simulink model "Rm1"  (Simulink 7.8)
settings: Solver=FixedStepDiscrete  StartTime=0.0  StopTime=10.0  RelTol=1e-3  SampleTimeConstraint=STIndependent
libraries: ApplFwS1v1_LIB x5
settings Model: Creator=z0035ypc  LastModifiedBy=z003019m
settings OptimizationCC: BooleanDataType=off  InlineParams=on
settings DebuggingCC: InheritedTsInSrcMsg=none  UnconnectedInputMsg=none  UnconnectedOutputMsg=none

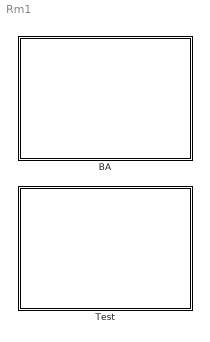
== system Rm1 ==
  BA : Subsystem
      mask Display: disp ('BA-Model');
  Test : Subsystem
      mask Display: disp ('Chart');

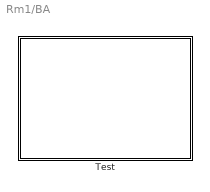
== system Rm1/BA ==
  Test : Subsystem
      mask Display: disp ('ViewNode Function');

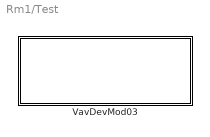
== system Rm1/Test ==
  VavDevMod03 : Subsystem
      mask Display: plot([0.5,0.5],[0.05,0.9]);text(0.5, 0.95,'VavDevMod03', 'HorizontalAlignment','center','VerticalAlignment','middle')

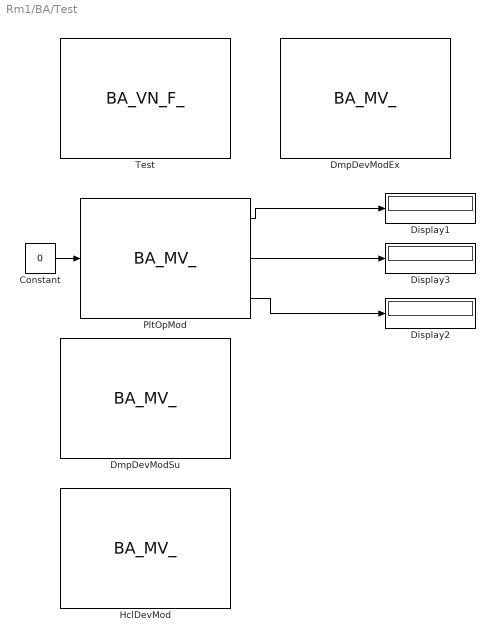
== system Rm1/BA/Test ==
  Constant : Constant  Value=0
  Display1 : Display
  Display2 : Display
  Display3 : Display
  DmpDevModEx : ApplFwS1v1_LIB/BA_OBJECT/BA_MV_  DefValue=1  NumOfStates=5  DeviceId=4194303  ObjectId=79691783
  DmpDevModSu : ApplFwS1v1_LIB/BA_OBJECT/BA_MV_  DefValue=1  NumOfStates=5  DeviceId=4194303  ObjectId=79691784
  HclDevMod : ApplFwS1v1_LIB/BA_OBJECT/BA_MV_  DefValue=1  NumOfStates=4  DeviceId=4194303  ObjectId=79691787
  PltOpMod : ApplFwS1v1_LIB/BA_OBJECT/BA_MV_  DefValue=1  NumOfStates=17  DeviceId=4194303  ObjectId=79691786
  Test : ApplFwS1v1_LIB/BA_OBJECT/BA_VN_F_  ItemDeviceId=[4194303 4194303 4194303 4194303]  ItemObjectId=[79691786 79691784 79691787 79691783]  DeviceId=[4194303]  ObjectId=[121634820]
  wires:
  PltOpMod/1 -> Display1/1
  PltOpMod/3 -> Display2/1
  PltOpMod/2 -> Display3/1
  Constant/1 -> PltOpMod/1

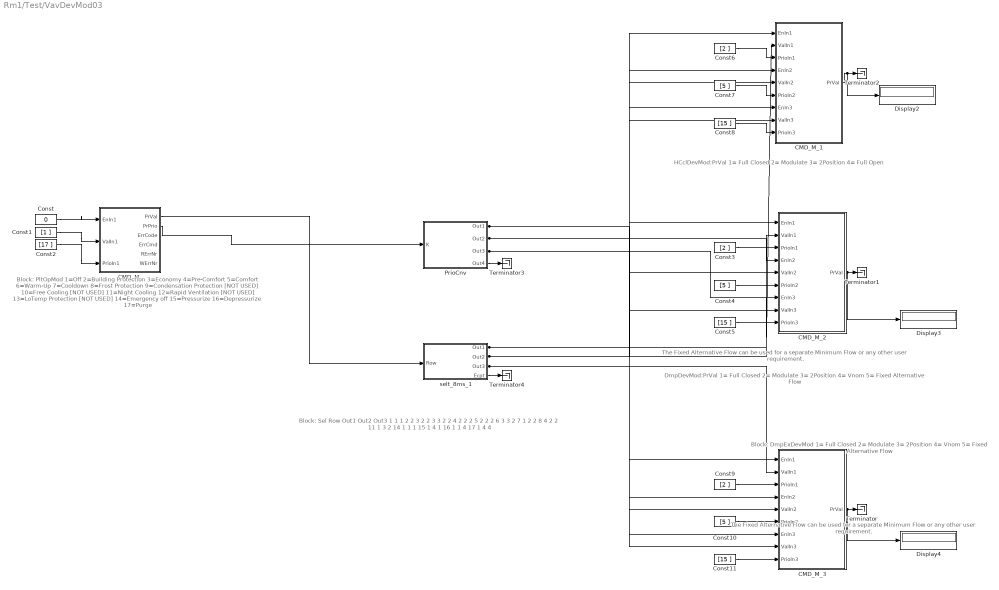
== system Rm1/Test/VavDevMod03 ==
  note: The Fixed Alternative Flow can be used for a separate Minimum Flow or any other user requirement.
  note: DmpDevMod:PrVal
      | 1= Full Closed
      | 2= Modulate
      | 3= 2Position
      | 4= Vnom
      | 5= Fixed Alternative Flow
  note: HCclDevMod:PrVal
      | 1= Full Closed
      | 2= Modulate
      | 3= 2Position
      | 4= Full Open
  note: Block: PltOpMod
      |
      | 1=Off
      | 2=Building Protection
      | 3=Economy
      | 4=Pre-Comfort
      | 5=Comfort
      | 6=Warm-Up
      | 7=Cooldown
      | 8=Frost Protection
      | 9=Condensation Protection [NOT USED]
      | 10=Free Cooling [NOT USED]
      | 11=Night Cooling
      | 12=Rapid Ventilation [NOT USED]
      | 13=LoTemp Protection [NOT USED]
      | 14=Emergency off
      | 15=Pressurize
      | 16=Depressurize
      | 17=Purge
  note: Block: Sel
      | Row  Out1  Out2   Out3
      | 1         1         1          2
      | 2         3         2          2
      | 3         3         2          2
      | 4         2         2          2
      | 5         2         2          2
      | 6         3         3          2
      | 7         1         2          2
      | 8         4         2          2
      | 11       1         3          2
      | 14       1         1          1
      | 15       1         4          1
      | 16       1         1          4
      | 17       1         4          4
  note: The Fixed Alternative Flow can be used for a separate Minimum Flow or any other user requirement.
  note: Block: DmpExDevMod
      | 1= Full Closed
      | 2= Modulate
      | 3= 2Position
      | 4= Vnom
      | 5= Fixed Alternative Flow
  CMD_M_ : Subsystem  mask{Invisible_1=off, Invisible_2=off, Invisible_3=off, Invisible_4=on, Invisible_5=on, Invisible_6=on, Invisible_7=on, Invisible_8=on, Invisible_9=on, Invisible_10=on, Invisible_11=on, Invisible_12=on, Invisible_13=on, Invisible_14=on, Invisible_15=on, Invisible_16=on, Invisible_17=off, Invisible_18=on, Invisible_19=off, Invisible_20=off, Invisible_21=off, Invisible_22=off, Invisible_23=off, Default_EnIn1=0, Default_ValIn1=0, Default_PrioIn1=0, Default_RptcIn1=0, Default_EnIn2=0, Default_ValIn2=0, Default_PrioIn2=0, Default_RptcIn2=0, Default_EnIn3=0, Default_ValIn3=0, Default_PrioIn3=0, Default_RptcIn3=0, Default_EnIn4=0, Default_ValIn4=0, Default_PrioIn4=0, Default_RptcIn4=0, DeviceId=4194303, ObjectId=121634820, ItemId=1, '=}
      mask prompts: Invisible_1 "EnIn1: Invisible"; Invisible_2 "ValIn1: Invisible"; Invisible_3 "PrioIn1: Invisible"; Invisible_4 "RptcIn1: Invisible"; Invisible_5 "EnIn2: Invisible"; Invisible_6 "ValIn2: Invisible"; Invisible_7 "PrioIn2: Invisible"; Invisible_8 "RptcIn2: Invisible"; Invisible_9 "EnIn3: Invisible"; Invisible_10 "ValIn3: Invisible"; Invisible_11 "PrioIn3: Invisible"; Invisible_12 "RptcIn3: Invisible"; Invisible_13 "EnIn4: Invisible"; Invisible_14 "ValIn4: Invisible"; Invisible_15 "PrioIn4: Invisible"; Invisible_16 "RptcIn4: Invisible"; Invisible_17 "PrVal: Invisible"; Invisible_18 "Valid: Invisible"; Invisible_19 "PrPrio: Invisible"; Invisible_20 "ErrCode: Invisible"; Invisible_21 "ErrCmd: Invisible"; Invisible_22 "RErrNr: Invisible"; Invisible_23 "WErrNr: Invisible"; Default_EnIn1 "EnIn1: Default"; Default_ValIn1 "ValIn1: Default"; Default_PrioIn1 "PrioIn1: Default"; Default_RptcIn1 "RptcIn1: Default"; Default_EnIn2 "EnIn2: Default"; Default_ValIn2 "ValIn2: Default"; Default_PrioIn2 "PrioIn2: Default"; Default_RptcIn2 "RptcIn2: Default"; Default_EnIn3 "EnIn3: Default"; Default_ValIn3 "ValIn3: Default"; Default_PrioIn3 "PrioIn3: Default"; Default_RptcIn3 "RptcIn3: Default"; Default_EnIn4 "EnIn4: Default"; Default_ValIn4 "ValIn4: Default"; Default_PrioIn4 "PrioIn4: Default"; Default_RptcIn4 "RptcIn4: Default"; DeviceId "BaObjRef.DeviceId"; ObjectId "BaObjRef.ObjectId"; ItemId "BaObjRef.ItemId"
      mask Help: web(['file:///' which('SiemensBuildingLibraryHelp0deDE.chm')])
      mask CallbackString: Callback(1)|Callback(2)|Callback(3)|Callback(4)|Callback(5)|Callback(6)|Callback(7)|Callback(8)|Callback(9)|Callback(10)|Callback(11)|Callback(12)|Callback(13)|Callback(14)|Callback(15)|Callback(16)|Callback(17)|Callback(18)|Callback(19)|Callback(20)|Callback(21)|Callback(22)|Callback(23)|Callback(24)|Callback(25)|Callback(26)|Callback(27)|Callback(28)|Callback(29)|Callback(30)|Callback(31)|Callback(32)|Callback(33)|Callback(34)|Callback(35)|Callback(36)|Callback(37)|Callback(38)|Callback(39)|||
      mask Display:
      | plot([0.5,0.5],[0,0.9])
      | text(0.5, 0.95,' CMD_M ', 'HorizontalAlignment', 'center')
  CMD_M_1 : Subsystem  mask{Invisible_1=off, Invisible_2=off, Invisible_3=off, Invisible_4=on, Invisible_5=off, Invisible_6=off, Invisible_7=off, Invisible_8=on, Invisible_9=off, Invisible_10=off, Invisible_11=off, Invisible_12=on, Invisible_13=on, Invisible_14=on, Invisible_15=on, Invisible_16=on, Invisible_17=off, Invisible_18=on, Invisible_19=on, Invisible_20=on, Invisible_21=on, Invisible_22=on, Invisible_23=on, Default_EnIn1=0, Default_ValIn1=0, Default_PrioIn1=0, Default_RptcIn1=0, Default_EnIn2=0, Default_ValIn2=0, Default_PrioIn2=0, Default_RptcIn2=0, Default_EnIn3=0, Default_ValIn3=0, Default_PrioIn3=0, Default_RptcIn3=0, Default_EnIn4=0, Default_ValIn4=0, Default_PrioIn4=0, Default_RptcIn4=0, DeviceId=4194303, ObjectId=121634820, ItemId=3, '=}
      mask prompts: Invisible_1 "EnIn1: Invisible"; Invisible_2 "ValIn1: Invisible"; Invisible_3 "PrioIn1: Invisible"; Invisible_4 "RptcIn1: Invisible"; Invisible_5 "EnIn2: Invisible"; Invisible_6 "ValIn2: Invisible"; Invisible_7 "PrioIn2: Invisible"; Invisible_8 "RptcIn2: Invisible"; Invisible_9 "EnIn3: Invisible"; Invisible_10 "ValIn3: Invisible"; Invisible_11 "PrioIn3: Invisible"; Invisible_12 "RptcIn3: Invisible"; Invisible_13 "EnIn4: Invisible"; Invisible_14 "ValIn4: Invisible"; Invisible_15 "PrioIn4: Invisible"; Invisible_16 "RptcIn4: Invisible"; Invisible_17 "PrVal: Invisible"; Invisible_18 "Valid: Invisible"; Invisible_19 "PrPrio: Invisible"; Invisible_20 "ErrCode: Invisible"; Invisible_21 "ErrCmd: Invisible"; Invisible_22 "RErrNr: Invisible"; Invisible_23 "WErrNr: Invisible"; Default_EnIn1 "EnIn1: Default"; Default_ValIn1 "ValIn1: Default"; Default_PrioIn1 "PrioIn1: Default"; Default_RptcIn1 "RptcIn1: Default"; Default_EnIn2 "EnIn2: Default"; Default_ValIn2 "ValIn2: Default"; Default_PrioIn2 "PrioIn2: Default"; Default_RptcIn2 "RptcIn2: Default"; Default_EnIn3 "EnIn3: Default"; Default_ValIn3 "ValIn3: Default"; Default_PrioIn3 "PrioIn3: Default"; Default_RptcIn3 "RptcIn3: Default"; Default_EnIn4 "EnIn4: Default"; Default_ValIn4 "ValIn4: Default"; Default_PrioIn4 "PrioIn4: Default"; Default_RptcIn4 "RptcIn4: Default"; DeviceId "BaObjRef.DeviceId"; ObjectId "BaObjRef.ObjectId"; ItemId "BaObjRef.ItemId"
      mask Help: web(['file:///' which('SiemensBuildingLibraryHelp0deDE.chm')])
      mask CallbackString: Callback(1)|Callback(2)|Callback(3)|Callback(4)|Callback(5)|Callback(6)|Callback(7)|Callback(8)|Callback(9)|Callback(10)|Callback(11)|Callback(12)|Callback(13)|Callback(14)|Callback(15)|Callback(16)|Callback(17)|Callback(18)|Callback(19)|Callback(20)|Callback(21)|Callback(22)|Callback(23)|Callback(24)|Callback(25)|Callback(26)|Callback(27)|Callback(28)|Callback(29)|Callback(30)|Callback(31)|Callback(32)|Callback(33)|Callback(34)|Callback(35)|Callback(36)|Callback(37)|Callback(38)|Callback(39)|||
      mask Display:
      | plot([0.5,0.5],[0,0.9])
      | text(0.5, 0.95,' CMD_M ', 'HorizontalAlignment', 'center')
  CMD_M_2 : Subsystem  mask{Invisible_1=off, Invisible_2=off, Invisible_3=off, Invisible_4=on, Invisible_5=off, Invisible_6=off, Invisible_7=off, Invisible_8=on, Invisible_9=off, Invisible_10=off, Invisible_11=off, Invisible_12=on, Invisible_13=on, Invisible_14=on, Invisible_15=on, Invisible_16=on, Invisible_17=off, Invisible_18=on, Invisible_19=on, Invisible_20=on, Invisible_21=on, Invisible_22=on, Invisible_23=on, Default_EnIn1=0, Default_ValIn1=0, Default_PrioIn1=0, Default_RptcIn1=0, Default_EnIn2=0, Default_ValIn2=0, Default_PrioIn2=0, Default_RptcIn2=0, Default_EnIn3=0, Default_ValIn3=0, Default_PrioIn3=0, Default_RptcIn3=0, Default_EnIn4=0, Default_ValIn4=0, Default_PrioIn4=0, Default_RptcIn4=0, DeviceId=4194303, ObjectId=121634820, ItemId=2, '=}
      mask prompts: Invisible_1 "EnIn1: Invisible"; Invisible_2 "ValIn1: Invisible"; Invisible_3 "PrioIn1: Invisible"; Invisible_4 "RptcIn1: Invisible"; Invisible_5 "EnIn2: Invisible"; Invisible_6 "ValIn2: Invisible"; Invisible_7 "PrioIn2: Invisible"; Invisible_8 "RptcIn2: Invisible"; Invisible_9 "EnIn3: Invisible"; Invisible_10 "ValIn3: Invisible"; Invisible_11 "PrioIn3: Invisible"; Invisible_12 "RptcIn3: Invisible"; Invisible_13 "EnIn4: Invisible"; Invisible_14 "ValIn4: Invisible"; Invisible_15 "PrioIn4: Invisible"; Invisible_16 "RptcIn4: Invisible"; Invisible_17 "PrVal: Invisible"; Invisible_18 "Valid: Invisible"; Invisible_19 "PrPrio: Invisible"; Invisible_20 "ErrCode: Invisible"; Invisible_21 "ErrCmd: Invisible"; Invisible_22 "RErrNr: Invisible"; Invisible_23 "WErrNr: Invisible"; Default_EnIn1 "EnIn1: Default"; Default_ValIn1 "ValIn1: Default"; Default_PrioIn1 "PrioIn1: Default"; Default_RptcIn1 "RptcIn1: Default"; Default_EnIn2 "EnIn2: Default"; Default_ValIn2 "ValIn2: Default"; Default_PrioIn2 "PrioIn2: Default"; Default_RptcIn2 "RptcIn2: Default"; Default_EnIn3 "EnIn3: Default"; Default_ValIn3 "ValIn3: Default"; Default_PrioIn3 "PrioIn3: Default"; Default_RptcIn3 "RptcIn3: Default"; Default_EnIn4 "EnIn4: Default"; Default_ValIn4 "ValIn4: Default"; Default_PrioIn4 "PrioIn4: Default"; Default_RptcIn4 "RptcIn4: Default"; DeviceId "BaObjRef.DeviceId"; ObjectId "BaObjRef.ObjectId"; ItemId "BaObjRef.ItemId"
      mask Help: web(['file:///' which('SiemensBuildingLibraryHelp0deDE.chm')])
      mask CallbackString: Callback(1)|Callback(2)|Callback(3)|Callback(4)|Callback(5)|Callback(6)|Callback(7)|Callback(8)|Callback(9)|Callback(10)|Callback(11)|Callback(12)|Callback(13)|Callback(14)|Callback(15)|Callback(16)|Callback(17)|Callback(18)|Callback(19)|Callback(20)|Callback(21)|Callback(22)|Callback(23)|Callback(24)|Callback(25)|Callback(26)|Callback(27)|Callback(28)|Callback(29)|Callback(30)|Callback(31)|Callback(32)|Callback(33)|Callback(34)|Callback(35)|Callback(36)|Callback(37)|Callback(38)|Callback(39)|||
      mask Display:
      | plot([0.5,0.5],[0,0.9])
      | text(0.5, 0.95,' CMD_M ', 'HorizontalAlignment', 'center')
  CMD_M_3 : Subsystem  mask{Invisible_1=off, Invisible_2=off, Invisible_3=off, Invisible_4=on, Invisible_5=off, Invisible_6=off, Invisible_7=off, Invisible_8=on, Invisible_9=off, Invisible_10=off, Invisible_11=off, Invisible_12=on, Invisible_13=on, Invisible_14=on, Invisible_15=on, Invisible_16=on, Invisible_17=off, Invisible_18=on, Invisible_19=on, Invisible_20=on, Invisible_21=on, Invisible_22=on, Invisible_23=on, Default_EnIn1=0, Default_ValIn1=0, Default_PrioIn1=0, Default_RptcIn1=0, Default_EnIn2=0, Default_ValIn2=0, Default_PrioIn2=0, Default_RptcIn2=0, Default_EnIn3=0, Default_ValIn3=0, Default_PrioIn3=0, Default_RptcIn3=0, Default_EnIn4=0, Default_ValIn4=0, Default_PrioIn4=0, Default_RptcIn4=0, DeviceId=4194303, ObjectId=121634820, ItemId=4, '=}
      mask prompts: Invisible_1 "EnIn1: Invisible"; Invisible_2 "ValIn1: Invisible"; Invisible_3 "PrioIn1: Invisible"; Invisible_4 "RptcIn1: Invisible"; Invisible_5 "EnIn2: Invisible"; Invisible_6 "ValIn2: Invisible"; Invisible_7 "PrioIn2: Invisible"; Invisible_8 "RptcIn2: Invisible"; Invisible_9 "EnIn3: Invisible"; Invisible_10 "ValIn3: Invisible"; Invisible_11 "PrioIn3: Invisible"; Invisible_12 "RptcIn3: Invisible"; Invisible_13 "EnIn4: Invisible"; Invisible_14 "ValIn4: Invisible"; Invisible_15 "PrioIn4: Invisible"; Invisible_16 "RptcIn4: Invisible"; Invisible_17 "PrVal: Invisible"; Invisible_18 "Valid: Invisible"; Invisible_19 "PrPrio: Invisible"; Invisible_20 "ErrCode: Invisible"; Invisible_21 "ErrCmd: Invisible"; Invisible_22 "RErrNr: Invisible"; Invisible_23 "WErrNr: Invisible"; Default_EnIn1 "EnIn1: Default"; Default_ValIn1 "ValIn1: Default"; Default_PrioIn1 "PrioIn1: Default"; Default_RptcIn1 "RptcIn1: Default"; Default_EnIn2 "EnIn2: Default"; Default_ValIn2 "ValIn2: Default"; Default_PrioIn2 "PrioIn2: Default"; Default_RptcIn2 "RptcIn2: Default"; Default_EnIn3 "EnIn3: Default"; Default_ValIn3 "ValIn3: Default"; Default_PrioIn3 "PrioIn3: Default"; Default_RptcIn3 "RptcIn3: Default"; Default_EnIn4 "EnIn4: Default"; Default_ValIn4 "ValIn4: Default"; Default_PrioIn4 "PrioIn4: Default"; Default_RptcIn4 "RptcIn4: Default"; DeviceId "BaObjRef.DeviceId"; ObjectId "BaObjRef.ObjectId"; ItemId "BaObjRef.ItemId"
      mask Help: web(['file:///' which('SiemensBuildingLibraryHelp0deDE.chm')])
      mask CallbackString: Callback(1)|Callback(2)|Callback(3)|Callback(4)|Callback(5)|Callback(6)|Callback(7)|Callback(8)|Callback(9)|Callback(10)|Callback(11)|Callback(12)|Callback(13)|Callback(14)|Callback(15)|Callback(16)|Callback(17)|Callback(18)|Callback(19)|Callback(20)|Callback(21)|Callback(22)|Callback(23)|Callback(24)|Callback(25)|Callback(26)|Callback(27)|Callback(28)|Callback(29)|Callback(30)|Callback(31)|Callback(32)|Callback(33)|Callback(34)|Callback(35)|Callback(36)|Callback(37)|Callback(38)|Callback(39)|||
      mask Display:
      | plot([0.5,0.5],[0,0.9])
      | text(0.5, 0.95,' CMD_M ', 'HorizontalAlignment', 'center')
  Const : Constant  Value=0  SampleTime=-1
  Const1 : Constant  Value=[1 ]  SampleTime=-1
  Const10 : Constant  Value=[5 ]  SampleTime=-1
  Const11 : Constant  Value=[15 ]  SampleTime=-1
  Const2 : Constant  Value=[17 ]  SampleTime=-1
  Const3 : Constant  Value=[2 ]  SampleTime=-1
  Const4 : Constant  Value=[5 ]  SampleTime=-1
  Const5 : Constant  Value=[15 ]  SampleTime=-1
  Const6 : Constant  Value=[2 ]  SampleTime=-1
  Const7 : Constant  Value=[5 ]  SampleTime=-1
  Const8 : Constant  Value=[15 ]  SampleTime=-1
  Const9 : Constant  Value=[2 ]  SampleTime=-1
  Display2 : Display
  Display3 : Display
  Display4 : Display
  PrioCnv : Subsystem  AncestorBlock=ApplFwS1v1_LIB/CONVERT/PRIO_CNV_  mask{Invisible_1=off, Invisible_2=on, Invisible_3=on, Invisible_4=on, Invisible_5=on, Invisible_6=on, Invisible_7=on, Invisible_8=on, Invisible_9=on, Invisible_10=on, Invisible_11=on, Invisible_12=on, Invisible_13=on, Invisible_14=on, Invisible_15=on, Invisible_16=on, Invisible_17=on, Invisible_18=on, Invisible_19=off, Invisible_20=off, Invisible_21=off, Invisible_22=off, Default_K=0, Default_Prio1=1, Default_Prio2=1, Default_Prio3=1, Default_Prio4=2, Default_Prio5=2, Default_Prio6=2, Default_Prio7=3, Default_Prio8=3, Default_Prio9=3, Default_Prio10=3, Default_Prio11=3, Default_Prio12=3, Default_Prio13=3, Default_Prio14=3, Default_Prio15=3, Default_Prio16=3, Default_Prio17=3, '=}
      mask prompts: Invisible_1 "K: Invisible"; Invisible_2 "Prio1: Invisible"; Invisible_3 "Prio2: Invisible"; Invisible_4 "Prio3: Invisible"; Invisible_5 "Prio4: Invisible"; Invisible_6 "Prio5: Invisible"; Invisible_7 "Prio6: Invisible"; Invisible_8 "Prio7: Invisible"; Invisible_9 "Prio8: Invisible"; Invisible_10 "Prio9: Invisible"; Invisible_11 "Prio10: Invisible"; Invisible_12 "Prio11: Invisible"; Invisible_13 "Prio12: Invisible"; Invisible_14 "Prio13: Invisible"; Invisible_15 "Prio14: Invisible"; Invisible_16 "Prio15: Invisible"; Invisible_17 "Prio16: Invisible"; Invisible_18 "Prio17: Invisible"; Invisible_19 "Out1: Invisible"; Invisible_20 "Out2: Invisible"; Invisible_21 "Out3: Invisible"; Invisible_22 "Out4: Invisible"; Default_K "K: Default"; Default_Prio1 "Prio1: Default"; Default_Prio2 "Prio2: Default"; Default_Prio3 "Prio3: Default"; Default_Prio4 "Prio4: Default"; Default_Prio5 "Prio5: Default"; Default_Prio6 "Prio6: Default"; Default_Prio7 "Prio7: Default"; Default_Prio8 "Prio8: Default"; Default_Prio9 "Prio9: Default"; Default_Prio10 "Prio10: Default"; Default_Prio11 "Prio11: Default"; Default_Prio12 "Prio12: Default"; Default_Prio13 "Prio13: Default"; Default_Prio14 "Prio14: Default"; Default_Prio15 "Prio15: Default"; Default_Prio16 "Prio16: Default"; Default_Prio17 "Prio17: Default"
      mask Help: web(['file:///' which('SiemensBuildingLibraryHelp0deDE.chm')])
      mask CallbackString: Callback(1)|Callback(2)|Callback(3)|Callback(4)|Callback(5)|Callback(6)|Callback(7)|Callback(8)|Callback(9)|Callback(10)|Callback(11)|Callback(12)|Callback(13)|Callback(14)|Callback(15)|Callback(16)|Callback(17)|Callback(18)|Callback(19)|Callback(20)|Callback(21)|Callback(22)|Callback(23)|Callback(24)|Callback(25)|Callback(26)|Callback(27)|Callback(28)|Callback(29)|Callback(30)|Callback(31)|Callback(32)|Callback(33)|Callback(34)|Callback(35)|Callback(36)|Callback(37)|Callback(38)|Callback(39)|Callback(40)
      mask Display:
      | plot([0.5,0.5],[0,0.9])
      | text(0.5, 0.95,' PRIO_CNV ', 'HorizontalAlignment', 'center')
  Terminator{,1..4} (5 alike) : Terminator
  selt_8ms_1 : Subsystem  AncestorBlock=ApplFwS1v1_LIB/MULTIPLX/SELT_8MS_  mask{Invisible_1=off, Invisible_2=on, Invisible_3=on, Invisible_4=on, Invisible_5=on, Invisible_6=on, Invisible_7=on, Invisible_8=on, Invisible_9=on, Invisible_10=on, Invisible_11=on, Invisible_12=on, Invisible_13=on, Invisible_14=on, Invisible_15=on, Invisible_16=on, Invisible_17=on, Invisible_18=on, Invisible_19=on, Invisible_20=on, Invisible_21=on, Invisible_22=on, Invisible_23=on, Invisible_24=on, Invisible_25=on, Invisible_26=on, Invisible_27=on, Invisible_28=off, Invisible_29=off, Invisible_30=off, Invisible_31=on, Invisible_32=on, Invisible_33=on, Invisible_34=on, Invisible_35=on, Invisible_36=off, Invisible_37=on, Default_Row=0, Default_RowCnd=[ 1 2 3 4 5 6 7 8 9 10 11 12 13 14 15 16 17 18 19 20 21 22 23 24 ], Default_ValRow1=[ 1 1 2 1 1 1 1 1 ], Default_ValRow2=[ 3 2 2 1 1 1 1 1 ], Default_ValRow3=[ 3 2 2 1 1 1 1 1 ], Default_ValRow4=[ 2 2 2 1 1 1 1 1 ], Default_ValRow5=[ 2 2 2 1 1 1 1 1 ], Default_ValRow6=[ 3 3 2 1 1 1 1 1 ], Default_ValRow7=[ 1 2 2 1 1 1 1 1 ], Default_ValRow8=[ 4 2 2 1 1 1 1 1 ], Default_ValRow9=[ 1 1 1 1 1 1 1 1 ], Default_ValRow10=[ 1 1 1 1 1 1 1 1 ], Default_ValRow11=[ 1 3 2 1 1 1 1 1 ], Default_ValRow12=[ 1 1 1 1 1 1 1 1 ], Default_ValRow13=[ 1 1 1 1 1 1 1 1 ], Default_ValRow14=[ 1 1 1 1 1 1 1 1 ], Default_ValRow15=[ 1 4 1 1 1 1 1 1 ], Default_ValRow16=[ 1 1 4 1 1 1 1 1 ], Default_ValRow17=[ 1 4 4 1 1 1 1 1 ], Default_ValRow18=[ 1 1 1 1 1 1 1 1 ], Default_ValRow19=[ 1 1 1 1 1 1 1 1 ], Default_ValRow20=[ 1 1 1 1 1 1 1 1 ], Default_ValRow21=[ 1 1 1 1 1 1 1 1 ], Default_ValRow22=[ 1 1 1 1 1 1 1 1 ], Default_ValRow23=[ 1 1 1 1 1 1 1 1 ], Default_ValRow24=[ 1 1 1 1 1 1 1 1 ], Default_EcptVal=1}
      mask prompts: Invisible_1 "Row: Invisible"; Invisible_2 "RowCnd: Invisible"; Invisible_3 "ValRow1: Invisible"; Invisible_4 "ValRow2: Invisible"; Invisible_5 "ValRow3: Invisible"; Invisible_6 "ValRow4: Invisible"; Invisible_7 "ValRow5: Invisible"; Invisible_8 "ValRow6: Invisible"; Invisible_9 "ValRow7: Invisible"; Invisible_10 "ValRow8: Invisible"; Invisible_11 "ValRow9: Invisible"; Invisible_12 "ValRow10: Invisible"; Invisible_13 "ValRow11: Invisible"; Invisible_14 "ValRow12: Invisible"; Invisible_15 "ValRow13: Invisible"; Invisible_16 "ValRow14: Invisible"; Invisible_17 "ValRow15: Invisible"; Invisible_18 "ValRow16: Invisible"; Invisible_19 "ValRow17: Invisible"; Invisible_20 "ValRow18: Invisible"; Invisible_21 "ValRow19: Invisible"; Invisible_22 "ValRow20: Invisible"; Invisible_23 "ValRow21: Invisible"; Invisible_24 "ValRow22: Invisible"; Invisible_25 "ValRow23: Invisible"; Invisible_26 "ValRow24: Invisible"; Invisible_27 "EcptVal: Invisible"; Invisible_28 "Out1: Invisible"; Invisible_29 "Out2: Invisible"; Invisible_30 "Out3: Invisible"; Invisible_31 "Out4: Invisible"; Invisible_32 "Out5: Invisible"; Invisible_33 "Out6: Invisible"; Invisible_34 "Out7: Invisible"; Invisible_35 "Out8: Invisible"; Invisible_36 "EcptActv: Invisible"; Invisible_37 "DataBlkItf: Invisible"; Default_Row "Row: Default"; Default_RowCnd "RowCnd: Default"; Default_ValRow1 "ValRow1: Default"; Default_ValRow2 "ValRow2: Default"; Default_ValRow3 "ValRow3: Default"; Default_ValRow4 "ValRow4: Default"; Default_ValRow5 "ValRow5: Default"; Default_ValRow6 "ValRow6: Default"; Default_ValRow7 "ValRow7: Default"; Default_ValRow8 "ValRow8: Default"; Default_ValRow9 "ValRow9: Default"; Default_ValRow10 "ValRow10: Default"; Default_ValRow11 "ValRow11: Default"; Default_ValRow12 "ValRow12: Default"; Default_ValRow13 "ValRow13: Default"; Default_ValRow14 "ValRow14: Default"; Default_ValRow15 "ValRow15: Default"; Default_ValRow16 "ValRow16: Default"; Default_ValRow17 "ValRow17: Default"; Default_ValRow18 "ValRow18: Default"; Default_ValRow19 "ValRow19: Default"; Default_ValRow20 "ValRow20: Default"; Default_ValRow21 "ValRow21: Default"; Default_ValRow22 "ValRow22: Default"; Default_ValRow23 "ValRow23: Default"; Default_ValRow24 "ValRow24: Default"; Default_EcptVal "EcptVal: Default"
      mask Help: web(['file:///' which('SiemensBuildingLibraryHelp0deDE.chm')])
      mask CallbackString: Callback(1)|Callback(2)|Callback(3)|Callback(4)|Callback(5)|Callback(6)|Callback(7)|Callback(8)|Callback(9)|Callback(10)|Callback(11)|Callback(12)|Callback(13)|Callback(14)|Callback(15)|Callback(16)|Callback(17)|Callback(18)|Callback(19)|Callback(20)|Callback(21)|Callback(22)|Callback(23)|Callback(24)|Callback(25)|Callback(26)|Callback(27)|Callback(28)|Callback(29)|Callback(30)|Callback(31)|Callback(32)|Callback(33)|Callback(34)|Callback(35)|Callback(36)|Callback(37)|Callback(38)|Callback(39)|Callback(40)|Callback(41)|Callback(42)|Callback(43)|Callback(44)|Callback(45)|Callback(46)|Callback(47)|Callback(48)|Callback(49)|Callback(50)|Callback(51)|Callback(52)|Callback(53)|Callback(54)|Callback(55)|Callback(56)|Callback(57)|Callback(58)|Callback(59)|Callback(60)|Callback(61)|Callback(62)|Callback(63)|Callback(64)
      mask Display:
      | plot([0.5,0.5],[0,0.9])
      | text(0.5, 0.95,' SELT_8MS ', 'HorizontalAlignment', 'center')
  wires:
  Const/1 -> CMD_M_/1(EnIn1)
  Const1/1 -> CMD_M_/2(ValIn1)
  Const2/1 -> CMD_M_/3(PrioIn1)
  Const3/1 -> CMD_M_2/3(PrioIn1)
  Const4/1 -> CMD_M_2/6(PrioIn2)
  Const5/1 -> CMD_M_2/9(PrioIn3)
  Const6/1 -> CMD_M_1/3(PrioIn1)
  Const7/1 -> CMD_M_1/6(PrioIn2)
  Const8/1 -> CMD_M_1/9(PrioIn3)
  Const9/1 -> CMD_M_3/3(PrioIn1)
  Const10/1 -> CMD_M_3/6(PrioIn2)
  Const11/1 -> CMD_M_3/9(PrioIn3)
  CMD_M_/1(PrVal) -> selt_8ms_1/1(Row)
  CMD_M_/2(PrPrio) -> PrioCnv/1(K)
  PrioCnv/1(Out1) -> CMD_M_1/1(EnIn1), CMD_M_2/1(EnIn1), CMD_M_3/1(EnIn1)
  PrioCnv/2(Out2) -> CMD_M_1/4(EnIn2), CMD_M_2/4(EnIn2), CMD_M_3/4(EnIn2)
  PrioCnv/3(Out3) -> CMD_M_1/7(EnIn3), CMD_M_2/7(EnIn3), CMD_M_3/7(EnIn3)
  selt_8ms_1/1(Out1) -> CMD_M_1/8(ValIn3), CMD_M_1/5(ValIn2), CMD_M_1/2(ValIn1)
  selt_8ms_1/2(Out2) -> CMD_M_2/8(ValIn3), CMD_M_2/5(ValIn2), CMD_M_2/2(ValIn1)
  selt_8ms_1/3(Out3) -> CMD_M_3/8(ValIn3), CMD_M_3/5(ValIn2), CMD_M_3/2(ValIn1)
  CMD_M_3/1(PrVal) -> Terminator/1, Display4/1
  CMD_M_2/1(PrVal) -> Terminator1/1, Display3/1
  CMD_M_1/1(PrVal) -> Terminator2/1, Display2/1
  PrioCnv/4(Out4) -> Terminator3/1
  selt_8ms_1/4(Ecpt) -> Terminator4/1

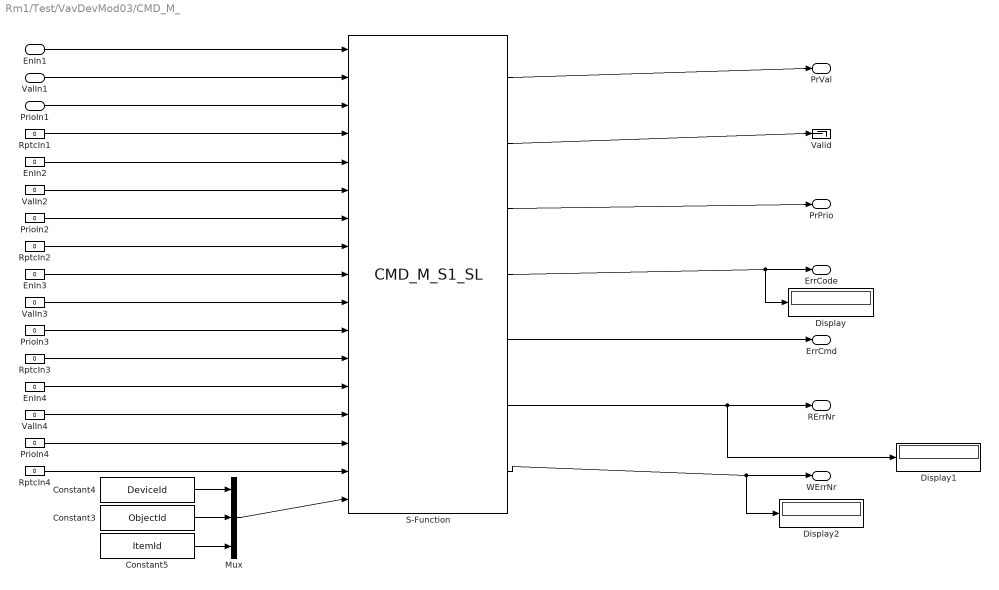
== system Rm1/Test/VavDevMod03/CMD_M_ ==
  EnIn1 : Inport
  ValIn1 : Inport  Port=2
  PrioIn1 : Inport  Port=3
  Constant3 : Constant  Value=ObjectId  OutDataTypeStr=Inherit: Inherit via back propagation  SampleTime=-1
  Constant4 : Constant  Value=DeviceId  OutDataTypeStr=Inherit: Inherit via back propagation  SampleTime=-1
  Constant5 : Constant  Value=ItemId  OutDataTypeStr=Inherit: Inherit via back propagation  SampleTime=-1
  Display : Display
  Display1 : Display
  Display2 : Display
  EnIn2 : Constant  Value=0  SampleTime=-1
  EnIn3 : Constant  Value=0  SampleTime=-1
  EnIn4 : Constant  Value=0  SampleTime=-1
  Mux : Mux  Inputs=3
  PrioIn2 : Constant  Value=0  SampleTime=-1
  PrioIn3 : Constant  Value=0  SampleTime=-1
  PrioIn4 : Constant  Value=0  SampleTime=-1
  RptcIn{1..4} (4 alike) : Constant  Value=0  SampleTime=-1
  S-Function : S-Function  FunctionName=CMD_M_S1_SL  Parameters=-1  EnableBusSupport=off
  ValIn2 : Constant  Value=0  SampleTime=-1
  ValIn3 : Constant  Value=0  SampleTime=-1
  ValIn4 : Constant  Value=0  SampleTime=-1
  Valid : Terminator
  PrVal : Outport
  PrPrio : Outport  Port=2
  ErrCode : Outport  Port=3
  ErrCmd : Outport  Port=4
  RErrNr : Outport  Port=5
  WErrNr : Outport  Port=6
  wires:
  EnIn1/1 -> S-Function/1
  ValIn1/1 -> S-Function/2
  PrioIn1/1 -> S-Function/3
  RptcIn1/1 -> S-Function/4
  EnIn2/1 -> S-Function/5
  ValIn2/1 -> S-Function/6
  PrioIn2/1 -> S-Function/7
  RptcIn2/1 -> S-Function/8
  EnIn3/1 -> S-Function/9
  ValIn3/1 -> S-Function/10
  PrioIn3/1 -> S-Function/11
  RptcIn3/1 -> S-Function/12
  EnIn4/1 -> S-Function/13
  ValIn4/1 -> S-Function/14
  PrioIn4/1 -> S-Function/15
  RptcIn4/1 -> S-Function/16
  Constant4/1 -> Mux/1
  Constant3/1 -> Mux/2
  Constant5/1 -> Mux/3
  Mux/1 -> S-Function/17
  S-Function/1 -> PrVal/1
  S-Function/2 -> Valid/1
  S-Function/3 -> PrPrio/1
  S-Function/4 -> ErrCode/1, Display/1
  S-Function/5 -> ErrCmd/1
  S-Function/6 -> Display1/1, RErrNr/1
  S-Function/7 -> WErrNr/1, Display2/1

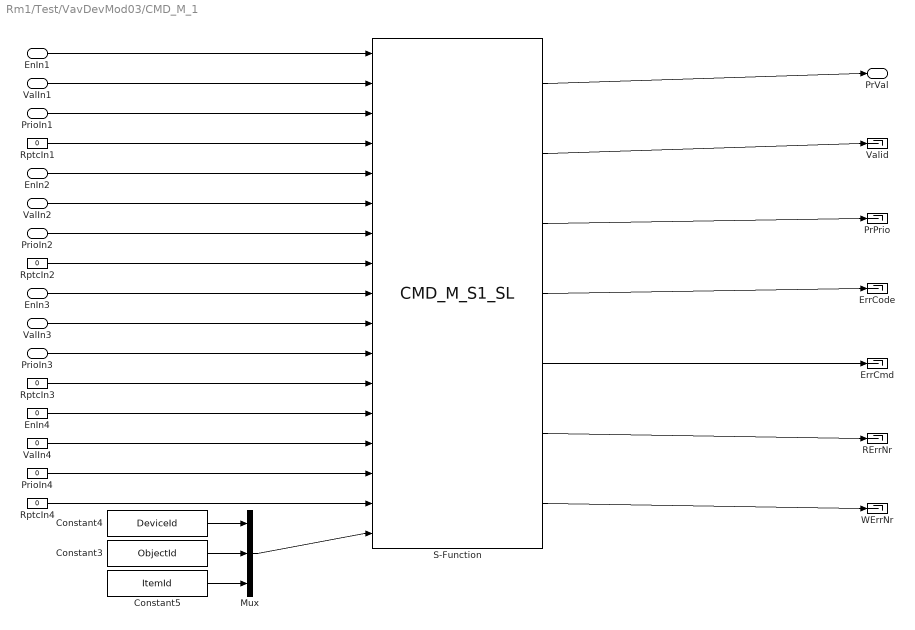
== system Rm1/Test/VavDevMod03/CMD_M_1 ==
  EnIn1 : Inport
  ValIn1 : Inport  Port=2
  PrioIn1 : Inport  Port=3
  EnIn2 : Inport  Port=4
  ValIn2 : Inport  Port=5
  PrioIn2 : Inport  Port=6
  EnIn3 : Inport  Port=7
  ValIn3 : Inport  Port=8
  PrioIn3 : Inport  Port=9
  Constant3 : Constant  Value=ObjectId  OutDataTypeStr=Inherit: Inherit via back propagation  SampleTime=-1
  Constant4 : Constant  Value=DeviceId  OutDataTypeStr=Inherit: Inherit via back propagation  SampleTime=-1
  Constant5 : Constant  Value=ItemId  OutDataTypeStr=Inherit: Inherit via back propagation  SampleTime=-1
  EnIn4 : Constant  Value=0  SampleTime=-1
  ErrCmd : Terminator
  ErrCode : Terminator
  Mux : Mux  Inputs=3
  PrPrio : Terminator
  PrioIn4 : Constant  Value=0  SampleTime=-1
  RErrNr : Terminator
  RptcIn{1..4} (4 alike) : Constant  Value=0  SampleTime=-1
  S-Function : S-Function  FunctionName=CMD_M_S1_SL  Parameters=-1  EnableBusSupport=off
  ValIn4 : Constant  Value=0  SampleTime=-1
  Valid : Terminator
  WErrNr : Terminator
  PrVal : Outport
  wires:
  EnIn1/1 -> S-Function/1
  ValIn1/1 -> S-Function/2
  PrioIn1/1 -> S-Function/3
  RptcIn1/1 -> S-Function/4
  EnIn2/1 -> S-Function/5
  ValIn2/1 -> S-Function/6
  PrioIn2/1 -> S-Function/7
  RptcIn2/1 -> S-Function/8
  EnIn3/1 -> S-Function/9
  ValIn3/1 -> S-Function/10
  PrioIn3/1 -> S-Function/11
  RptcIn3/1 -> S-Function/12
  EnIn4/1 -> S-Function/13
  ValIn4/1 -> S-Function/14
  PrioIn4/1 -> S-Function/15
  RptcIn4/1 -> S-Function/16
  Constant4/1 -> Mux/1
  Constant3/1 -> Mux/2
  Constant5/1 -> Mux/3
  Mux/1 -> S-Function/17
  S-Function/1 -> PrVal/1
  S-Function/2 -> Valid/1
  S-Function/3 -> PrPrio/1
  S-Function/4 -> ErrCode/1
  S-Function/5 -> ErrCmd/1
  S-Function/6 -> RErrNr/1
  S-Function/7 -> WErrNr/1

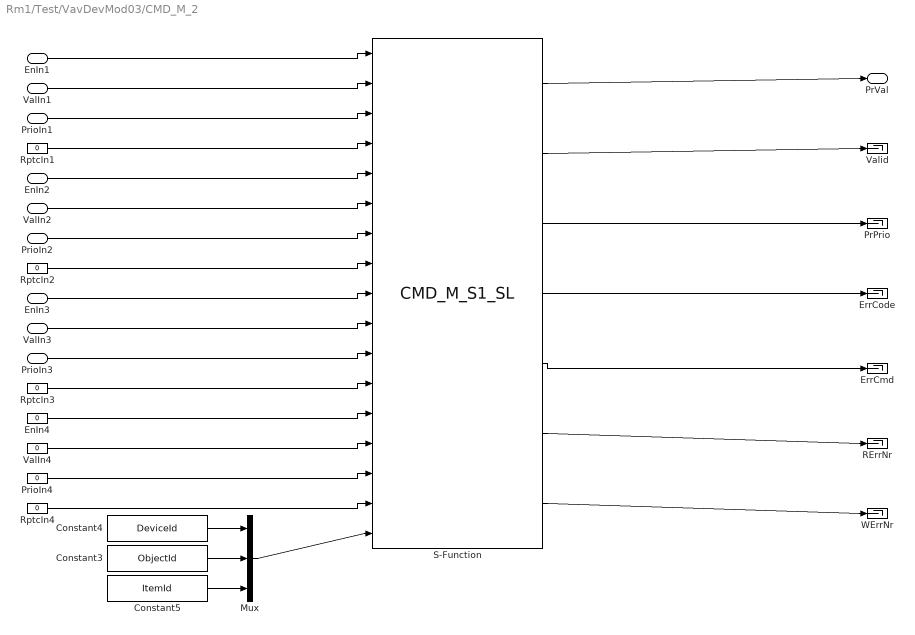
== system Rm1/Test/VavDevMod03/CMD_M_2 ==
  EnIn1 : Inport
  ValIn1 : Inport  Port=2
  PrioIn1 : Inport  Port=3
  EnIn2 : Inport  Port=4
  ValIn2 : Inport  Port=5
  PrioIn2 : Inport  Port=6
  EnIn3 : Inport  Port=7
  ValIn3 : Inport  Port=8
  PrioIn3 : Inport  Port=9
  Constant3 : Constant  Value=ObjectId  OutDataTypeStr=Inherit: Inherit via back propagation  SampleTime=-1
  Constant4 : Constant  Value=DeviceId  OutDataTypeStr=Inherit: Inherit via back propagation  SampleTime=-1
  Constant5 : Constant  Value=ItemId  OutDataTypeStr=Inherit: Inherit via back propagation  SampleTime=-1
  EnIn4 : Constant  Value=0  SampleTime=-1
  ErrCmd : Terminator
  ErrCode : Terminator
  Mux : Mux  Inputs=3
  PrPrio : Terminator
  PrioIn4 : Constant  Value=0  SampleTime=-1
  RErrNr : Terminator
  RptcIn{1..4} (4 alike) : Constant  Value=0  SampleTime=-1
  S-Function : S-Function  FunctionName=CMD_M_S1_SL  Parameters=-1  EnableBusSupport=off
  ValIn4 : Constant  Value=0  SampleTime=-1
  Valid : Terminator
  WErrNr : Terminator
  PrVal : Outport
  wires:
  EnIn1/1 -> S-Function/1
  ValIn1/1 -> S-Function/2
  PrioIn1/1 -> S-Function/3
  RptcIn1/1 -> S-Function/4
  EnIn2/1 -> S-Function/5
  ValIn2/1 -> S-Function/6
  PrioIn2/1 -> S-Function/7
  RptcIn2/1 -> S-Function/8
  EnIn3/1 -> S-Function/9
  ValIn3/1 -> S-Function/10
  PrioIn3/1 -> S-Function/11
  RptcIn3/1 -> S-Function/12
  EnIn4/1 -> S-Function/13
  ValIn4/1 -> S-Function/14
  PrioIn4/1 -> S-Function/15
  RptcIn4/1 -> S-Function/16
  Constant4/1 -> Mux/1
  Constant3/1 -> Mux/2
  Constant5/1 -> Mux/3
  Mux/1 -> S-Function/17
  S-Function/1 -> PrVal/1
  S-Function/2 -> Valid/1
  S-Function/3 -> PrPrio/1
  S-Function/4 -> ErrCode/1
  S-Function/5 -> ErrCmd/1
  S-Function/6 -> RErrNr/1
  S-Function/7 -> WErrNr/1

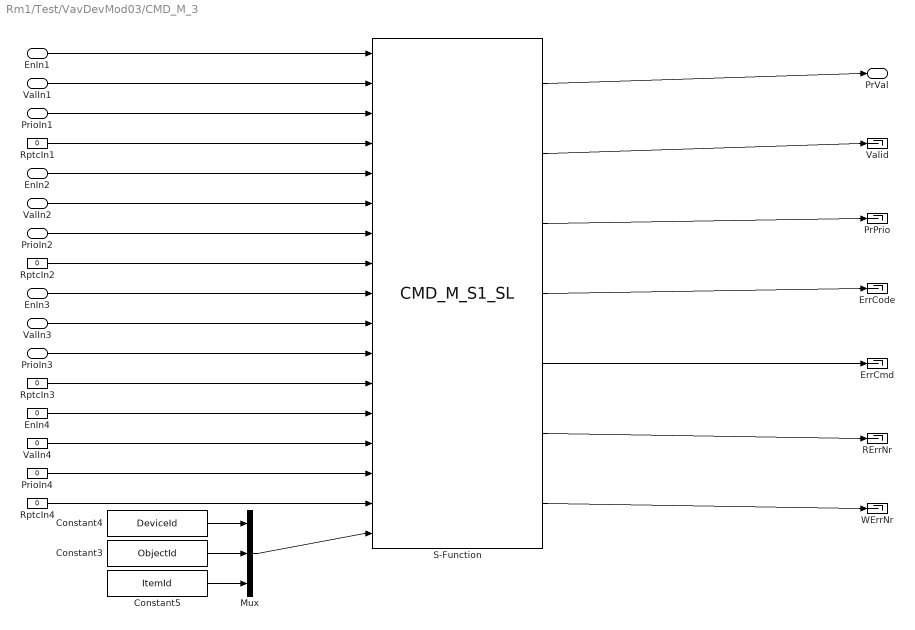
== system Rm1/Test/VavDevMod03/CMD_M_3 ==
  EnIn1 : Inport
  ValIn1 : Inport  Port=2
  PrioIn1 : Inport  Port=3
  EnIn2 : Inport  Port=4
  ValIn2 : Inport  Port=5
  PrioIn2 : Inport  Port=6
  EnIn3 : Inport  Port=7
  ValIn3 : Inport  Port=8
  PrioIn3 : Inport  Port=9
  Constant3 : Constant  Value=ObjectId  OutDataTypeStr=Inherit: Inherit via back propagation  SampleTime=-1
  Constant4 : Constant  Value=DeviceId  OutDataTypeStr=Inherit: Inherit via back propagation  SampleTime=-1
  Constant5 : Constant  Value=ItemId  OutDataTypeStr=Inherit: Inherit via back propagation  SampleTime=-1
  EnIn4 : Constant  Value=0  SampleTime=-1
  ErrCmd : Terminator
  ErrCode : Terminator
  Mux : Mux  Inputs=3
  PrPrio : Terminator
  PrioIn4 : Constant  Value=0  SampleTime=-1
  RErrNr : Terminator
  RptcIn{1..4} (4 alike) : Constant  Value=0  SampleTime=-1
  S-Function : S-Function  FunctionName=CMD_M_S1_SL  Parameters=-1  EnableBusSupport=off
  ValIn4 : Constant  Value=0  SampleTime=-1
  Valid : Terminator
  WErrNr : Terminator
  PrVal : Outport
  wires:
  EnIn1/1 -> S-Function/1
  ValIn1/1 -> S-Function/2
  PrioIn1/1 -> S-Function/3
  RptcIn1/1 -> S-Function/4
  EnIn2/1 -> S-Function/5
  ValIn2/1 -> S-Function/6
  PrioIn2/1 -> S-Function/7
  RptcIn2/1 -> S-Function/8
  EnIn3/1 -> S-Function/9
  ValIn3/1 -> S-Function/10
  PrioIn3/1 -> S-Function/11
  RptcIn3/1 -> S-Function/12
  EnIn4/1 -> S-Function/13
  ValIn4/1 -> S-Function/14
  PrioIn4/1 -> S-Function/15
  RptcIn4/1 -> S-Function/16
  Constant4/1 -> Mux/1
  Constant3/1 -> Mux/2
  Constant5/1 -> Mux/3
  Mux/1 -> S-Function/17
  S-Function/1 -> PrVal/1
  S-Function/2 -> Valid/1
  S-Function/3 -> PrPrio/1
  S-Function/4 -> ErrCode/1
  S-Function/5 -> ErrCmd/1
  S-Function/6 -> RErrNr/1
  S-Function/7 -> WErrNr/1

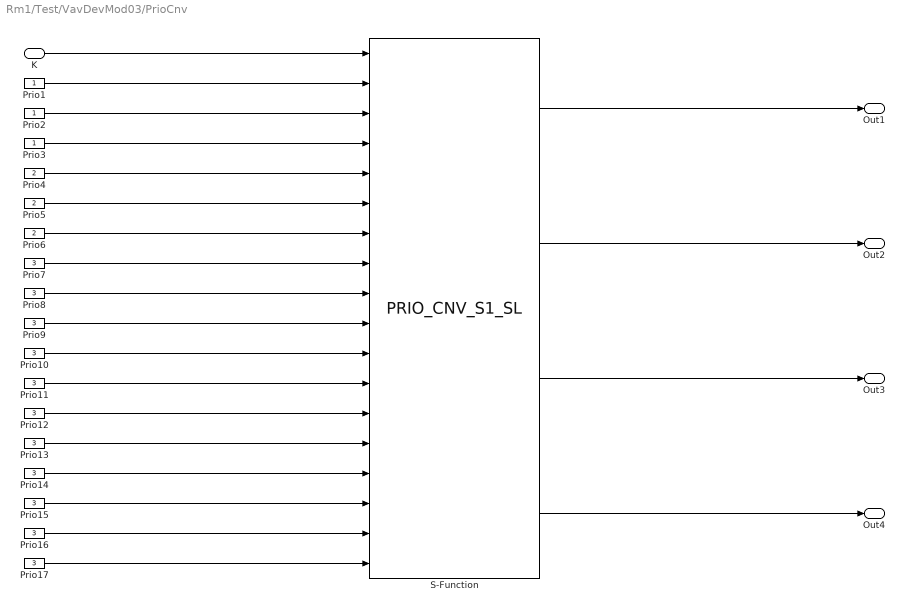
== system Rm1/Test/VavDevMod03/PrioCnv ==
  K : Inport
  Prio1 : Constant  SampleTime=-1
  Prio{7..17} (11 alike) : Constant  Value=3  SampleTime=-1
  Prio2 : Constant  SampleTime=-1
  Prio3 : Constant  SampleTime=-1
  Prio4 : Constant  Value=2  SampleTime=-1
  Prio5 : Constant  Value=2  SampleTime=-1
  Prio6 : Constant  Value=2  SampleTime=-1
  S-Function : S-Function  FunctionName=PRIO_CNV_S1_SL  Parameters=-1  EnableBusSupport=off
  Out1 : Outport
  Out2 : Outport  Port=2
  Out3 : Outport  Port=3
  Out4 : Outport  Port=4
  wires:
  S-Function/4 -> Out4/1
  S-Function/3 -> Out3/1
  S-Function/2 -> Out2/1
  S-Function/1 -> Out1/1
  Prio17/1 -> S-Function/18
  Prio16/1 -> S-Function/17
  Prio15/1 -> S-Function/16
  Prio14/1 -> S-Function/15
  Prio13/1 -> S-Function/14
  Prio12/1 -> S-Function/13
  Prio11/1 -> S-Function/12
  Prio10/1 -> S-Function/11
  Prio9/1 -> S-Function/10
  Prio8/1 -> S-Function/9
  Prio7/1 -> S-Function/8
  Prio6/1 -> S-Function/7
  Prio5/1 -> S-Function/6
  Prio4/1 -> S-Function/5
  Prio3/1 -> S-Function/4
  Prio2/1 -> S-Function/3
  Prio1/1 -> S-Function/2
  K/1 -> S-Function/1

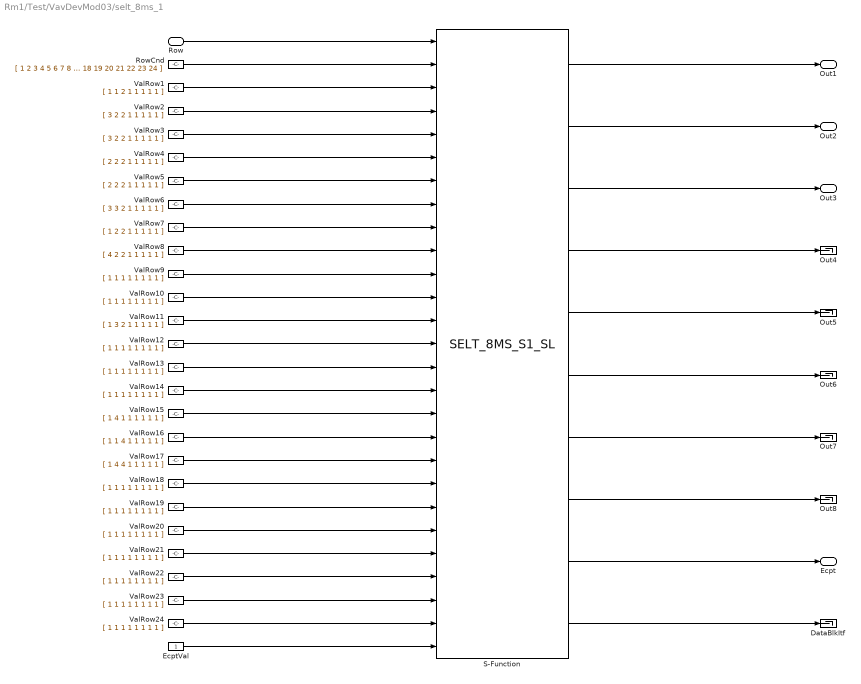
== system Rm1/Test/VavDevMod03/selt_8ms_1 ==
  Row : Inport
  DataBlkItf : Terminator
  EcptVal : Constant  SampleTime=-1
  Out{4..8} (5 alike) : Terminator
  RowCnd : Constant  Value=[ 1 2 3 4 5 6 7 8 9 10 11 12 13 14 15 16 17 18 19 20 21 22 23 24 ]  SampleTime=-1
  S-Function : S-Function  FunctionName=SELT_8MS_S1_SL  Parameters=-1  EnableBusSupport=off
  ValRow1 : Constant  Value=[ 1 1 2 1 1 1 1 1 ]  SampleTime=-1
  ValRow{9..10,12..14,18..24} (12 alike) : Constant  Value=[ 1 1 1 1 1 1 1 1 ]  SampleTime=-1
  ValRow11 : Constant  Value=[ 1 3 2 1 1 1 1 1 ]  SampleTime=-1
  ValRow15 : Constant  Value=[ 1 4 1 1 1 1 1 1 ]  SampleTime=-1
  ValRow16 : Constant  Value=[ 1 1 4 1 1 1 1 1 ]  SampleTime=-1
  ValRow17 : Constant  Value=[ 1 4 4 1 1 1 1 1 ]  SampleTime=-1
  ValRow2 : Constant  Value=[ 3 2 2 1 1 1 1 1 ]  SampleTime=-1
  ValRow3 : Constant  Value=[ 3 2 2 1 1 1 1 1 ]  SampleTime=-1
  ValRow4 : Constant  Value=[ 2 2 2 1 1 1 1 1 ]  SampleTime=-1
  ValRow5 : Constant  Value=[ 2 2 2 1 1 1 1 1 ]  SampleTime=-1
  ValRow6 : Constant  Value=[ 3 3 2 1 1 1 1 1 ]  SampleTime=-1
  ValRow7 : Constant  Value=[ 1 2 2 1 1 1 1 1 ]  SampleTime=-1
  ValRow8 : Constant  Value=[ 4 2 2 1 1 1 1 1 ]  SampleTime=-1
  Out1 : Outport
  Out2 : Outport  Port=2
  Out3 : Outport  Port=3
  Ecpt : Outport  Port=4
  wires:
  S-Function/10 -> DataBlkItf/1
  S-Function/9 -> Ecpt/1
  S-Function/8 -> Out8/1
  S-Function/7 -> Out7/1
  S-Function/6 -> Out6/1
  S-Function/5 -> Out5/1
  S-Function/4 -> Out4/1
  S-Function/3 -> Out3/1
  S-Function/2 -> Out2/1
  S-Function/1 -> Out1/1
  EcptVal/1 -> S-Function/27
  ValRow24/1 -> S-Function/26
  ValRow23/1 -> S-Function/25
  ValRow22/1 -> S-Function/24
  ValRow21/1 -> S-Function/23
  ValRow20/1 -> S-Function/22
  ValRow19/1 -> S-Function/21
  ValRow18/1 -> S-Function/20
  ValRow17/1 -> S-Function/19
  ValRow16/1 -> S-Function/18
  ValRow15/1 -> S-Function/17
  ValRow14/1 -> S-Function/16
  ValRow13/1 -> S-Function/15
  ValRow12/1 -> S-Function/14
  ValRow11/1 -> S-Function/13
  ValRow10/1 -> S-Function/12
  ValRow9/1 -> S-Function/11
  ValRow8/1 -> S-Function/10
  ValRow7/1 -> S-Function/9
  ValRow6/1 -> S-Function/8
  ValRow5/1 -> S-Function/7
  ValRow4/1 -> S-Function/6
  ValRow3/1 -> S-Function/5
  ValRow2/1 -> S-Function/4
  ValRow1/1 -> S-Function/3
  RowCnd/1 -> S-Function/2
  Row/1 -> S-Function/1
